simulink model "uz_pmsm_model_old_commit"  (R2023b)
settings: Solver=FixedStepAuto  StartTime=0.0  StopTime=0.05  RelTol=1e-3
PreLoadFcn:
  | uz_pmsm_model_init_parameter
PostLoadFcn:
  | % Import the data from Excel for a lookup table
  | FluxMapData = readtable('C:\Users\Philipp\ultrazohm\ultrazohm_sw\ip_cores\uz_pmsm_model\FluxMapData_2023-05-26_13-07-57.csv');
  | % Row indices for lookup table
  | d_current_in_d_axis = FluxMapData(8:27,1:end);
  | % Column indices for lookup table
  | q_current_in_d_axis = FluxMapData(29:48,1:end);
  | % Output values for lookup table
  | d_Flux_d_axis = FluxMapData(50:69,1:end);
values from neighbouring files (symbols this model uses):
  ad1 = ad_1(1)    [LUT_approx_methode2a.m]    (also in LUT_approx_methode2a_clean.m = ad_self(1); LUT_approx_methode_2a_FEM.m; fitting_parameter.mat = 0.03048394862; fitting_parameter_48V_SynRM.mat = 0.0218446789236)
  ad2 = ad_1(2)    [LUT_approx_methode2a.m]    (also in LUT_approx_methode2a_clean.m = ad_self(2); LUT_approx_methode_2a_FEM.m; fitting_parameter.mat = 0.0402440194669; fitting_parameter_48V_SynRM.mat = 0.015691946268)
  ad3 = ad_1(3)    [LUT_approx_methode2a.m]    (also in LUT_approx_methode2a_clean.m = ad_self(3); LUT_approx_methode_2a_FEM.m; fitting_parameter.mat = -16.4812001193; fitting_parameter_48V_SynRM.mat = 2.77465564774)
  ad4 = ad_3_6(1)    [LUT_approx_methode2a.m]    (also in LUT_approx_methode2a_clean.m = ad_4_6(1); LUT_approx_methode_2a_FEM.m; fitting_parameter.mat = 1.2964378241; fitting_parameter_48V_SynRM.mat = 0.0214529395212)
  ad5 = ad_3_6(2)    [LUT_approx_methode2a.m]    (also in LUT_approx_methode2a_clean.m = ad_4_6(2); LUT_approx_methode_2a_FEM.m; fitting_parameter.mat = 0.000618316734858; fitting_parameter_48V_SynRM.mat = 0.0128514742508)
  ad6 = ad_3_6(3)    [LUT_approx_methode2a.m]    (also in LUT_approx_methode2a_clean.m = ad_4_6(3); LUT_approx_methode_2a_FEM.m; fitting_parameter.mat = -12.2755860444; fitting_parameter_48V_SynRM.mat = 2.54408267654)
  aq1 = aq_1(1)    [LUT_approx_methode2a.m]    (also in LUT_approx_methode2a_clean.m = aq_self(1); LUT_approx_methode_2a_FEM.m; fitting_parameter.mat = 0.0048166705291; fitting_parameter_48V_SynRM.mat = 0.00205546577039)
  aq2 = aq_1(2)    [LUT_approx_methode2a.m]    (also in LUT_approx_methode2a_clean.m = aq_self(2); LUT_approx_methode_2a_FEM.m; fitting_parameter.mat = 0.171595255564; fitting_parameter_48V_SynRM.mat = 0.0602932843871)
  aq3 = aq_1(3)    [LUT_approx_methode2a.m]    (also in LUT_approx_methode2a_clean.m = aq_self(3); LUT_approx_methode_2a_FEM.m; fitting_parameter.mat = 0.000926293864031; fitting_parameter_48V_SynRM.mat = 4.42738872822e-05)
  aq4 = aq_3_6(1)    [LUT_approx_methode2a.m]    (also in LUT_approx_methode2a_clean.m = aq_4_6(1); LUT_approx_methode_2a_FEM.m; fitting_parameter.mat = 0.00500187099075; fitting_parameter_48V_SynRM.mat = 0.000698420875152)
  aq5 = aq_3_6(2)    [LUT_approx_methode2a.m]    (also in LUT_approx_methode2a_clean.m = aq_4_6(2); LUT_approx_methode_2a_FEM.m; fitting_parameter.mat = 0.17052123489; fitting_parameter_48V_SynRM.mat = 0.0493122483219)
  aq6 = aq_3_6(3)    [LUT_approx_methode2a.m]    (also in LUT_approx_methode2a_clean.m = aq_4_6(3); LUT_approx_methode_2a_FEM.m; fitting_parameter.mat = 0.00091860845; fitting_parameter_48V_SynRM.mat = 4.14644316065e-05)
  d_current_d_Flux = FluxMapData{1,1:20}    [uz_pmsm_model_init_parameter.m]
  d_current_q_Flux = FluxMapData{66,1:20}    [uz_pmsm_model_init_parameter.m]
  entkopplung_dynamic = false    [compare_simulation_to_measurement.m]    (also in uz_pmsm_model_init_parameter.m; uz_pmsm_model_init_parameter_clean.m)
  entkopplung_linear = true    [compare_simulation_to_measurement.m]    (also in uz_pmsm_model_init_parameter.m = false; uz_pmsm_model_init_parameter_clean.m = false)
  entkopplung_static = false    [compare_simulation_to_measurement.m]    (also in uz_pmsm_model_init_parameter.m = true; uz_pmsm_model_init_parameter_clean.m)
  Fid1_Giq1 = ((1/2).*(aq3-aq6).*((q_current_set).^2))+((aq1./aq2).*log(cosh(aq2.*q_current_set)))-((aq4/aq5).*log(cosh(aq5.*q_current_set)))    [LUT_approx_methode2a.m]    (also in LUT_approx_methode2a_clean.m; LUT_approx_methode_2a_FEM.m = (1/2).*(aq3-aq6).*((q_current_set).^2)+((aq1./aq2).*log(cosh; fitting_parameter.mat = -0.00135679401385; fitting_parameter_48V_SynRM.mat = 0.221350145237)
  Fid2_Giq2 = ((ad1./ad2).*(log(cosh(ad2.*(d_current_set-ad3))))) - ((ad4./ad5).*(log(cosh(ad5.*(d_current_set-ad6)))))    [LUT_approx_methode2a.m]    (also in LUT_approx_methode2a_clean.m; LUT_approx_methode_2a_FEM.m = ((ad1./ad2).*(log(cosh(ad2.*(d_current_set-ad3))))) - (((ad1; fitting_parameter.mat = 0.0788137932988; fitting_parameter_48V_SynRM.mat = 0.221214979406)
  Flux_d = FluxMapData{43:62,1:20}'*(1e-3)    [uz_pmsm_model_init_parameter.m]
  Flux_q = FluxMapData{108:127,1:20}'*(1e-3)    [uz_pmsm_model_init_parameter.m]
  friction_coefficient = 0.001    [uz_pmsm_model_init_parameter.m]    (also in uz_pmsm_model_init_parameter_clean.m)
  inertia = 0.000084    (= 8.4e-05)    [uz_pmsm_model_init_parameter.m]    (also in uz_pmsm_model_init_parameter_clean.m)
  L_d = 0.3    [uz_pmsm_model_init_parameter.m]    (also in uz_pmsm_model_init_parameter_clean.m = 0.00045)
  L_q = 0.3    [uz_pmsm_model_init_parameter.m]    (also in uz_pmsm_model_init_parameter_clean.m = 0.002)
  load_torque = 0    [uz_pmsm_model_init_parameter.m]
  parameter_nachfuerung = false    [compare_simulation_to_measurement.m]    (also in uz_pmsm_model_init_parameter.m; uz_pmsm_model_init_parameter_clean.m)
  polepair = 4    [uz_pmsm_model_init_parameter.m]    (also in uz_pmsm_model_init_parameter_clean.m)
  praediktion_entkopplung_nonlinear = false    [compare_simulation_to_measurement.m]    (also in uz_pmsm_model_init_parameter.m; uz_pmsm_model_init_parameter_clean.m = true)
  psi_pm = 0.0075    [uz_pmsm_model_init_parameter.m]    (also in uz_pmsm_model_init_parameter_clean.m = 0.0194)
  q_current_d_Flux = FluxMapData{22:41,1}    [uz_pmsm_model_init_parameter.m]
  q_current_q_Flux = FluxMapData{87:106,1}    [uz_pmsm_model_init_parameter.m]
  R_1 = 0.08    [uz_pmsm_model_init_parameter.m]    (also in uz_pmsm_model_init_parameter_clean.m = 0.3)
  rpm = 1250    [uz_pmsm_model_init_parameter.m]
  setpoint_step = 4.0    (= 4)    [compare_simulation_to_measurement.m]    (also in export_csv.m = 10; iae_von_cil_measurements.m = 8; uz_pmsm_model_init_parameter.m = 8; uz_pmsm_model_init_parameter_clean.m = 10)
  simulate_mechanical = true    [compare_simulation_to_measurement.m]    (also in export_csv.m = false; uz_pmsm_model_init_parameter.m = false; uz_pmsm_model_init_parameter_clean.m = false)
  simulate_nonlinear_modell = false    [compare_simulation_to_measurement.m]    (also in uz_pmsm_model_init_parameter.m = true; uz_pmsm_model_init_parameter_clean.m = true)
  simulate_open_loop = true    [compare_simulation_to_measurement.m]    (also in export_csv.m; uz_pmsm_model_init_parameter.m = false; uz_pmsm_model_init_parameter_clean.m = false)
  static_friction_torque = 0.01    [uz_pmsm_model_init_parameter.m]    (also in uz_pmsm_model_init_parameter_clean.m)
  tau_sum = 2*ts_regler    (= 0.0001)    [uz_pmsm_model_init_parameter.m]    (also in uz_pmsm_model_init_parameter_clean.m = 8e-05)
  ts = logs{k}.Values    [export_csv.m]    (also in uz_pmsm_model_init_parameter.m = 2e-06; uz_pmsm_model_init_parameter_clean.m = 2e-06)
  ts_regler = 1/20e3    (= 5e-05)    [uz_pmsm_model_init_parameter.m]    (also in uz_pmsm_model_init_parameter_clean.m = 4e-05)
undefined symbols (not defined in the file or in its folder): Ki_Bo_d, Ki_Bo_q, Kp_Bo_d, Kp_Bo_q, Ldq
libraries: slpidlib x6
(part 2 of 5)

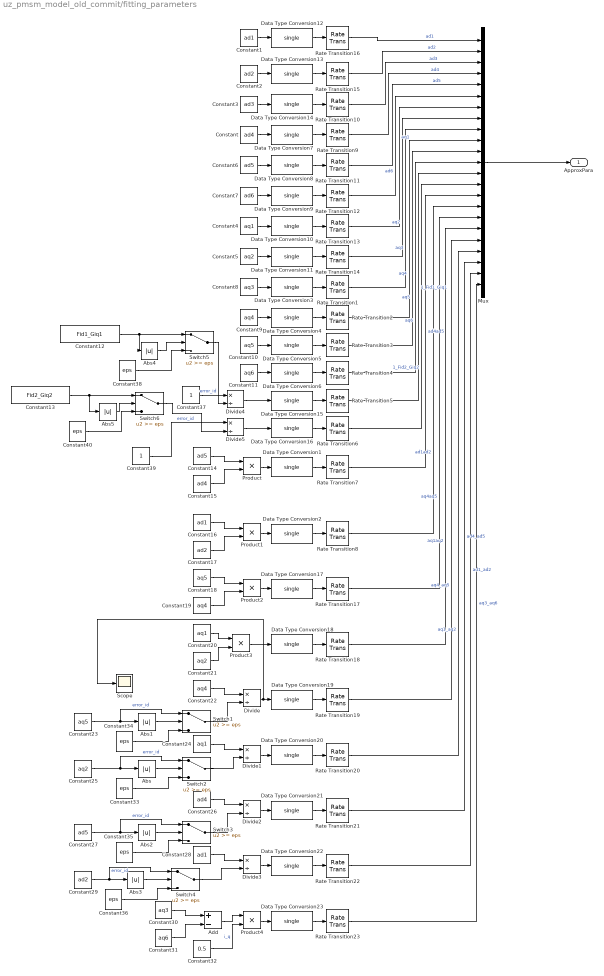
== system uz_pmsm_model_old_commit/fitting_parameters ==
  Abs{,1..5} (6 alike) : Abs  SaturateOnIntegerOverflow=off
  Add : Sum  Inputs=+-
  Constant : Constant  Value=ad4
  Constant1 : Constant  Value=ad1
  Constant10 : Constant  Value=aq5
  Constant11 : Constant  Value=aq6
  Constant12 : Constant  Value=Fid1_Giq1
  Constant13 : Constant  Value=Fid2_Giq2
  Constant14 : Constant  Value=ad5
  Constant15 : Constant  Value=ad4
  Constant16 : Constant  Value=ad1
  Constant17 : Constant  Value=ad2
  Constant18 : Constant  Value=aq5
  Constant19 : Constant  Value=aq4
  Constant2 : Constant  Value=ad2
  Constant20 : Constant  Value=aq1
  Constant21 : Constant  Value=aq2
  Constant22 : Constant  Value=aq4
  Constant23 : Constant  Value=aq5
  Constant24 : Constant  Value=aq1
  Constant25 : Constant  Value=aq2
  Constant26 : Constant  Value=ad4
  Constant27 : Constant  Value=ad5
  Constant28 : Constant  Value=ad1
  Constant29 : Constant  Value=ad2
  Constant3 : Constant  Value=ad3
  Constant30 : Constant  Value=aq3
  Constant31 : Constant  Value=aq6
  Constant32 : Constant  Value=0.5  OutDataTypeStr=double  SampleTime=-1
  Constant{33..36,38,40} (6 alike) : Constant  Value=eps  SampleTime=ts_regler
  Constant37 : Constant
  Constant39 : Constant
  Constant4 : Constant  Value=aq1
  Constant5 : Constant  Value=aq2
  Constant6 : Constant  Value=ad5
  Constant7 : Constant  Value=ad6
  Constant8 : Constant  Value=aq3
  Constant9 : Constant  Value=aq4
  Data Type Conversion{1..23} (23 alike) : DataTypeConversion  OutDataTypeStr=single  SaturateOnIntegerOverflow=off  RndMeth=Floor
  Divide{,1..5} (6 alike) : Product  Inputs=*/
  Mux : Mux  Inputs=23
  Product{,1..4} (5 alike) : Product
  Rate Transition{1..23} (23 alike) : RateTransition  OutPortSampleTime=ts
  Scope : Scope
  Switch{1..6} (6 alike) : Switch  Threshold=eps  SaturateOnIntegerOverflow=off  InputSameDT=off
  ApproxPara : Outport
  wires:
  Constant1/1 -> Data Type Conversion12/1
  Constant/1 -> Data Type Conversion7/1
  Rate Transition10/1 -> Mux/3  "ad3"
  Rate Transition14/1 -> Mux/8  "aq2"
  Constant3/1 -> Data Type Conversion14/1
  Rate Transition12/1 -> Mux/6  "ad6"
  Rate Transition16/1 -> Mux/1  "ad1"
  Rate Transition13/1 -> Mux/7  "aq1"
  Constant5/1 -> Data Type Conversion11/1
  Constant7/1 -> Data Type Conversion9/1
  Rate Transition15/1 -> Mux/2  "ad2"
  Rate Transition9/1 -> Mux/4  "ad4"
  Constant6/1 -> Data Type Conversion8/1
  Constant4/1 -> Data Type Conversion10/1
  Rate Transition11/1 -> Mux/5  "ad5"
  Constant2/1 -> Data Type Conversion13/1
  Rate Transition1/1 -> Mux/9  "aq3"
  Constant8/1 -> Data Type Conversion3/1
  Rate Transition2/1 -> Mux/10  "aq4"
  Constant9/1 -> Data Type Conversion4/1
  Rate Transition3/1 -> Mux/11  "aq5"
  Constant10/1 -> Data Type Conversion5/1
  Rate Transition4/1 -> Mux/12  "aq6"
  Constant11/1 -> Data Type Conversion6/1
  Rate Transition5/1 -> Mux/13  "1_Fid1_Giq1"
  Rate Transition6/1 -> Mux/14  "1_Fid2_Giq2"
  Data Type Conversion11/1 -> Rate Transition14/1
  Data Type Conversion10/1 -> Rate Transition13/1
  Data Type Conversion9/1 -> Rate Transition12/1
  Data Type Conversion12/1 -> Rate Transition16/1
  Data Type Conversion13/1 -> Rate Transition15/1
  Data Type Conversion14/1 -> Rate Transition10/1
  Data Type Conversion7/1 -> Rate Transition9/1
  Data Type Conversion8/1 -> Rate Transition11/1
  Data Type Conversion3/1 -> Rate Transition1/1
  Data Type Conversion4/1 -> Rate Transition2/1
  Data Type Conversion5/1 -> Rate Transition3/1
  Data Type Conversion6/1 -> Rate Transition4/1
  Data Type Conversion15/1 -> Rate Transition5/1
  Data Type Conversion16/1 -> Rate Transition6/1
  Constant14/1 -> Product/1
  Constant15/1 -> Product/2
  Product/1 -> Data Type Conversion1/1
  Data Type Conversion1/1 -> Rate Transition7/1
  Rate Transition7/1 -> Mux/15  "ad4ad5"
  Rate Transition8/1 -> Mux/16  "ad1ad2"
  Constant16/1 -> Product1/1
  Constant17/1 -> Product1/2
  Data Type Conversion2/1 -> Rate Transition8/1
  Product1/1 -> Data Type Conversion2/1
  Constant18/1 -> Product2/1
  Constant19/1 -> Product2/2
  Data Type Conversion17/1 -> Rate Transition17/1
  Product2/1 -> Data Type Conversion17/1
  Rate Transition18/1 -> Mux/18  "aq1aq2"
  Product3/1 -> Data Type Conversion18/1
  Data Type Conversion18/1 -> Rate Transition18/1
  Constant21/1 -> Product3/2
  Constant20/1 -> Product3/1
  Rate Transition17/1 -> Mux/17  "aq4aq5"
  Divide/1 -> Scope/1, Data Type Conversion19/1
  Data Type Conversion19/1 -> Rate Transition19/1
  Constant22/1 -> Divide/1
  Rate Transition19/1 -> Mux/19  "aq4_aq5"
  Constant24/1 -> Divide1/1
  Rate Transition20/1 -> Mux/20  "aq1_aq2"
  Divide1/1 -> Data Type Conversion20/1
  Data Type Conversion20/1 -> Rate Transition20/1
  Data Type Conversion21/1 -> Rate Transition21/1
  Divide2/1 -> Data Type Conversion21/1
  Rate Transition21/1 -> Mux/21  "ad4_ad5"
  Constant26/1 -> Divide2/1
  Constant28/1 -> Divide3/1
  Rate Transition22/1 -> Mux/22  "ad1_ad2"
  Divide3/1 -> Data Type Conversion22/1
  Data Type Conversion22/1 -> Rate Transition22/1
  Data Type Conversion23/1 -> Rate Transition23/1
  Constant30/1 -> Add/1
  Constant31/1 -> Add/2
  Rate Transition23/1 -> Mux/23  "aq3_aq6"
  Product4/1 -> Data Type Conversion23/1
  Constant32/1 -> Product4/2  "i_q"
  Add/1 -> Product4/1
  Mux/1 -> ApproxPara/1
  Constant25/1 -> Switch2/1, Abs/1  "error_id"
  Switch2/1 -> Divide1/2
  Abs/1 -> Switch2/2
  Constant33/1 -> Switch2/3
  Constant23/1 -> Switch1/1, Abs1/1  "error_id"
  Switch1/1 -> Divide/2
  Abs1/1 -> Switch1/2
  Constant34/1 -> Switch1/3
  Constant27/1 -> Switch3/1, Abs2/1  "error_id"
  Switch3/1 -> Divide2/2
  Abs2/1 -> Switch3/2
  Constant35/1 -> Switch3/3
  Constant29/1 -> Switch4/1, Abs3/1  "error_id"
  Switch4/1 -> Divide3/2
  Abs3/1 -> Switch4/2
  Constant36/1 -> Switch4/3
  Abs4/1 -> Switch5/2
  Constant38/1 -> Switch5/3
  Divide4/1 -> Data Type Conversion15/1
  Switch5/1 -> Divide4/2
  Constant12/1 -> Abs4/1, Switch5/1
  Constant37/1 -> Divide4/1  "error_id"
  Constant39/1 -> Divide5/1  "error_id"
  Constant13/1 -> Abs5/1, Switch6/1
  Constant40/1 -> Switch6/3
  Abs5/1 -> Switch6/2
  Divide5/1 -> Data Type Conversion16/1
  Switch6/1 -> Divide5/2

== system uz_pmsm_model_old_commit/model_parameters1 ==
  Bus Creator : BusCreator  Inputs=8
  Constant : Constant  Value=L_d
  Constant6 : Constant  Value=L_q
  Constant7 : Constant  Value=R_1
  Constant8 : Constant  Value=polepair
  Constant9 : Constant  Value=psi_pm
  Data Type Conversion{7..14} (8 alike) : DataTypeConversion  OutDataTypeStr=single  SaturateOnIntegerOverflow=off  RndMeth=Floor
  J : Constant  Value=1/inertia
  M_R0 : Constant  Value=static_friction_torque
  Rate Transition{9..16} (8 alike) : RateTransition  OutPortSampleTime=ts
  mu : Constant  Value=friction_coefficient
  Out1 : Outport
  wires:
  Data Type Conversion12/1 -> Rate Transition16/1
  Data Type Conversion7/1 -> Rate Transition9/1
  Rate Transition10/1 -> Bus Creator/3  "M_R0"
  Rate Transition14/1 -> Bus Creator/8  "psi_pm"
  Data Type Conversion14/1 -> Rate Transition10/1
  Rate Transition12/1 -> Bus Creator/6  "R_1"
  Rate Transition16/1 -> Bus Creator/1  "1_J"
  Rate Transition13/1 -> Bus Creator/7  "polepair"
  Bus Creator/1 -> Out1/1
  Data Type Conversion11/1 -> Rate Transition14/1
  Constant8/1 -> Data Type Conversion10/1
  Data Type Conversion9/1 -> Rate Transition12/1
  Rate Transition15/1 -> Bus Creator/2  "mu"
  Constant6/1 -> Data Type Conversion8/1
  Rate Transition9/1 -> Bus Creator/4  "1_L_d"
  J/1 -> Data Type Conversion12/1
  Data Type Conversion8/1 -> Rate Transition11/1
  Data Type Conversion10/1 -> Rate Transition13/1
  mu/1 -> Data Type Conversion13/1
  M_R0/1 -> Data Type Conversion14/1
  Rate Transition11/1 -> Bus Creator/5  "1_L_q"
  Data Type Conversion13/1 -> Rate Transition15/1
  Constant7/1 -> Data Type Conversion9/1
  Constant9/1 -> Data Type Conversion11/1
  Constant/1 -> Data Type Conversion7/1

== system uz_pmsm_model_old_commit/uz_pmsm_model ==
  reset_integrators : Inport
  simulate_mechanical : Inport  Port=2
  simulate_nonlinear : Inport  Port=3
  reciprocal_J : Inport  Port=4
  mu : Inport  Port=5
  M_n0 : Inport  Port=6
  R1 : Inport  Port=7
  polepairs : Inport  Port=8
  Ld : Inport  Port=9
  Lq : Inport  Port=10
  psi_pm : Inport  Port=11
  fitting_parameter : Inport  Port=12
  inputs : Inport  Port=13
  Demux : Demux
  Mux : Mux
  Switch : Switch  Criteria=u2 ~= 0  SaturateOnIntegerOverflow=off  InputSameDT=off
  Switch1 : Switch  Criteria=u2 ~= 0  SaturateOnIntegerOverflow=off  InputSameDT=off
  mechanical_system : Subsystem
  pmsm : Subsystem
  torque_calculation : Subsystem
  outputs : Outport
  wires:
  reset_integrators/1 -> pmsm/1(reset1), mechanical_system/1(reset)
  Demux/3 -> Switch1/3, Switch/3  "omega_mech"
  Switch/1 -> pmsm/11(omega_mech1)
  pmsm/2(psi_d1) -> torque_calculation/2(psi_d)
  Demux/4 -> mechanical_system/6(load_torque)  "load_torque"
  pmsm/3(psi_q1) -> torque_calculation/3(psi_q)
  Demux/1 -> pmsm/3(u_d1)  "u_d"
  simulate_mechanical/1 -> Switch1/2, Switch/2
  Demux/2 -> pmsm/4(u_q1)  "u_q"
  mechanical_system/1(omega_mech) -> Switch/1, Switch1/1
  pmsm/4(I_q1) -> torque_calculation/5(I_q), Mux/2  "i_q"
  pmsm/1(I_d1) -> Mux/1, torque_calculation/1(I_d)  "i_d"
  Switch1/1 -> Mux/4  "i_q"
  torque_calculation/1(M_Mi) -> mechanical_system/2(M_Mi), Mux/3  "i_q"
  inputs/1 -> Demux/1
  Mux/1 -> outputs/1
  simulate_nonlinear/1 -> pmsm/2(simulate_nonlinear)
  R1/1 -> pmsm/5(R2)
  polepairs/1 -> torque_calculation/4(polepairs), pmsm/6(polepairs1)
  Ld/1 -> pmsm/7(Ld)
  Lq/1 -> pmsm/8(Lq)
  psi_pm/1 -> pmsm/9(psi_pm)
  mu/1 -> mechanical_system/3(mu)
  M_n0/1 -> mechanical_system/4(M_n0)
  reciprocal_J/1 -> mechanical_system/5(reciprocal_J)
  fitting_parameter/1 -> pmsm/10(fitting_parameters)

== system uz_pmsm_model_old_commit/Curren t_Controller_With_FluxMaps_OLD/#embedded-Coder ==
  Psi_d_q : Subsystem
  Reglernachführung2 : Subsystem
  Subsystem : Subsystem
  approximate_flux_d : Subsystem
  approximate_flux_q : Subsystem

== system uz_pmsm_model_old_commit/Curren t_Controller_With_FluxMaps_OLD/Entkopplung_flags ==
  u_d_static : Inport
  u_q_static : Inport  Port=2
  u_d_praed : Inport  Port=3
  u_q_praed : Inport  Port=4
  u_d_lin : Inport  Port=5
  u_q_lin : Inport  Port=6
  u_d_dyn : Inport  Port=7
  u_q_dyn : Inport  Port=8
  0 : Constant  Value=0
  Switch{1..8} (8 alike) : Switch  Criteria=u2 > Threshold  SaturateOnIntegerOverflow=off  InputSameDT=off
  entkopplung_dynamic : Constant  Value=entkopplung_dynamic
  entkopplung_linear : Constant  Value=entkopplung_linear
  entkopplung_preadiktion : Constant  Value=praediktion_entkopplung_nonlinear
  entkopplung_static : Constant  Value=entkopplung_static
  u_d_entk : Outport
  u_q_entk : Outport  Port=2
  wires:
  Switch3/1 -> u_d_entk/1
  Switch4/1 -> Switch2/3
  entkopplung_preadiktion/1 -> Switch2/2, Switch3/2
  Switch1/1 -> Switch3/3
  u_d_praed/1 -> Switch3/1
  Switch2/1 -> u_q_entk/1
  u_q_praed/1 -> Switch2/1
  entkopplung_static/1 -> Switch4/2, Switch1/2
  u_d_static/1 -> Switch1/1
  u_d_lin/1 -> Switch5/1
  Switch5/1 -> Switch1/3
  entkopplung_linear/1 -> Switch6/2, Switch5/2
  entkopplung_dynamic/1 -> Switch8/2, Switch7/2
  0/1 -> Switch8/3, Switch7/3
  Switch6/1 -> Switch4/3
  u_q_static/1 -> Switch4/1
  u_q_lin/1 -> Switch6/1
  u_d_dyn/1 -> Switch7/1
  Switch8/1 -> Switch6/3
  u_q_dyn/1 -> Switch8/1
  Switch7/1 -> Switch5/3

== system uz_pmsm_model_old_commit/Curren t_Controller_With_FluxMaps_OLD/Entkopplungen ==
  u_q : Inport
  u_d : Inport  Port=2
  uq : Inport  Port=3
  ud : Inport  Port=4
  i_d : Inport  Port=5
  psi_d_LUT : Inport  Port=6
  psi_q_LUT : Inport  Port=7
  Ldq_LUT : Inport  Port=8
  Lqd_LUT : Inport  Port=9
  i_q : Inport  Port=10
  omega_m : Inport  Port=11
  Lineare_Entkopplung : Subsystem
  Scope : Scope  NumInputPorts=2
  decoupling_praediktion : Subsystem
  dynamic_nonlinear_entkopplung1 : Subsystem
  static_nonlinear_entkopplung : Subsystem
  u_d_static : Outport
  u_q_static : Outport  Port=2
  u_d_prae : Outport  Port=3
  u_q_prae : Outport  Port=4
  u_d_lin : Outport  Port=5
  u_q_lin : Outport  Port=6
  u_d_dyn : Outport  Port=7
  u_q_dyn1 : Outport  Port=8
  wires:
  psi_d_LUT/1 -> static_nonlinear_entkopplung/1(psi_d), dynamic_nonlinear_entkopplung1/3(psi_d), decoupling_praediktion/9(psi_d)
  omega_m/1 -> dynamic_nonlinear_entkopplung1/7(omega_m), Lineare_Entkopplung/3(omega_m), static_nonlinear_entkopplung/3(omega_m), decoupling_praediktion/5(omega_m)
  psi_q_LUT/1 -> dynamic_nonlinear_entkopplung1/4(psi_q), decoupling_praediktion/8(psi_q), static_nonlinear_entkopplung/2(psi_q)
  u_q/1 -> decoupling_praediktion/4(u_q_1)
  i_d/1 -> dynamic_nonlinear_entkopplung1/1(i_d), Lineare_Entkopplung/1(i_d), decoupling_praediktion/1(i_d)
  i_q/1 -> dynamic_nonlinear_entkopplung1/2(i_q), Lineare_Entkopplung/2(i_q), decoupling_praediktion/3(i_q)
  ud/1 -> decoupling_praediktion/6(u_d_k)
  uq/1 -> decoupling_praediktion/7(u_q_k)
  u_d/1 -> decoupling_praediktion/2(u_d_1)
  static_nonlinear_entkopplung/1(u_d) -> u_d_static/1
  Lineare_Entkopplung/1(u_d) -> Scope/1, u_d_lin/1
  static_nonlinear_entkopplung/2(u_q) -> u_q_static/1
  decoupling_praediktion/1(u_d_entk) -> u_d_prae/1
  Lineare_Entkopplung/2(u_q) -> Scope/2, u_q_lin/1
  decoupling_praediktion/2(u_q_entk) -> u_q_prae/1
  dynamic_nonlinear_entkopplung1/1(u_d) -> u_d_dyn/1
  dynamic_nonlinear_entkopplung1/2(u_q) -> u_q_dyn1/1
  Ldq_LUT/1 -> dynamic_nonlinear_entkopplung1/5(Ldq_LUT)
  Lqd_LUT/1 -> dynamic_nonlinear_entkopplung1/6(Lqd_LUT)

== system uz_pmsm_model_old_commit/Curren t_Controller_With_FluxMaps_OLD/Psi_d_q ==
  I_d_set : Inport
  I_d : Inport  Port=2
  I_q_set : Inport  Port=3
  I_q : Inport  Port=4
  ApproxPara : Inport  Port=5
  Constant4 : Constant  Value="eps(\"single\")"  SampleTime=ts_regler
  Constant5 : Constant  Value="eps(\"single\")"  SampleTime=ts_regler
  Data Type Conversion{1..5} (5 alike) : DataTypeConversion  OutDataTypeStr=single  SaturateOnIntegerOverflow=off  RndMeth=Floor
  Divide : Product  Inputs=*/
  Divide1 : Product  Inputs=*/
  Scope : Scope  NumInputPorts=4
  Sum{1..2,4..5} (4 alike) : Sum  Inputs=|+-
  Switch2 : Switch  Criteria=u2 ~= 0  Threshold=eps  SaturateOnIntegerOverflow=off  InputSameDT=off
  Switch3 : Switch  Criteria=u2 ~= 0  Threshold=eps  SaturateOnIntegerOverflow=off  InputSameDT=off
  psid_approx : Subsystem
  psid_approx1 : Subsystem
  psiq_approx : Subsystem
  psiq_approx1 : Subsystem
  Ldd_approx : Outport
  Lqq_approx : Outport  Port=2
  psid : Outport  Port=3
  psiq : Outport  Port=4
  wires:
  I_q/1 -> Data Type Conversion4/1
  psid_approx/1(psid) -> Scope/3, Sum4/1  "psi_d_set"
  psiq_approx/1(psiq) -> Scope/4, Sum5/1  "psi_q_set"
  ApproxPara/1 -> Data Type Conversion5/1
  I_d/1 -> Data Type Conversion2/1
  psiq_approx1/1(psiq) -> Scope/1, psiq/1, Sum5/2  "psi_q"
  psid_approx1/1(psid) -> Scope/2, psid/1, Sum4/2  "psi_d"
  Constant5/1 -> Switch3/3
  Switch2/1 -> Divide/2
  Switch3/1 -> Divide1/2
  Divide/1 -> Ldd_approx/1  "Ldd_approx"
  Divide1/1 -> Lqq_approx/1  "Lqq_approx"
  Constant4/1 -> Switch2/3
  Sum5/1 -> Divide1/1
  Sum4/1 -> Divide/1
  Sum2/1 -> Switch2/2, Switch2/1
  I_q_set/1 -> Data Type Conversion3/1
  I_d_set/1 -> Data Type Conversion1/1
  Sum1/1 -> Switch3/2, Switch3/1
  Data Type Conversion1/1 -> psid_approx/1(Id), Sum2/1  "omega_mech"
  Data Type Conversion3/1 -> Sum1/1, psiq_approx/2(Iq)  "omega_mech"
  Data Type Conversion2/1 -> psid_approx1/1(Id), psiq_approx1/1(Id), Sum2/2, psiq_approx/1(Id)  "omega_mech"
  Data Type Conversion4/1 -> Sum1/2, psiq_approx1/2(Iq), psid_approx1/2(Iq), psid_approx/2(Iq)  "omega_mech"
  Data Type Conversion5/1 -> psid_approx1/3(FittingParameters), psid_approx/3(FittingParameters), psiq_approx/3(FittingParameters), psiq_approx1/3(FittingParameters)  "omega_mech"

== system uz_pmsm_model_old_commit/Curren t_Controller_With_FluxMaps_OLD/Psi_d_q1 ==
  I_d : Inport
  I_q : Inport  Port=2
  ApproxPara : Inport  Port=3
  Ldd_approx1 : Subsystem
  Lqq_approx1 : Subsystem
  psid_approx : Subsystem
  psiq_approx : Subsystem
  psi_d : Outport
  Ldd : Outport  Port=2
  psi_q : Outport  Port=3
  Lqq : Outport  Port=4
  wires:
  psid_approx/1(psid) -> psi_d/1  "psi_d"
  psiq_approx/1(psiq) -> psi_q/1  "psi_q"
  I_q/1 -> psid_approx/2(Iq), Lqq_approx1/2(Iq), psiq_approx/2(Iq)
  psid_approx/2(psiq_cross_s1_integrated) -> Ldd_approx1/1(psiq_cross_s1_integrated)
  I_d/1 -> Ldd_approx1/2(Id), psid_approx/1(Id), psiq_approx/1(Id)
  psiq_approx/2(psid_cross_s1_integrated) -> Lqq_approx1/1(psid_cross_s1_integrated)
  Ldd_approx1/1(Ldd) -> Ldd/1  "Ldd"
  Lqq_approx1/1(Lqq) -> Lqq/1  "Lqq"
  ApproxPara/1 -> psiq_approx/3(FittingParameters), Ldd_approx1/3(FittingParameters), psid_approx/3(FittingParameters), Lqq_approx1/3(FittingParameters)

== system uz_pmsm_model_old_commit/Curren t_Controller_With_FluxMaps_OLD/Psi_d_q2 ==
  I_d_set : Inport
  I_d : Inport  Port=2
  I_q_set : Inport  Port=3
  I_q : Inport  Port=4
  ApproxPara : Inport  Port=5
  Ldd_approx1 : Subsystem
  Lqq_approx1 : Subsystem
  Scope : Scope  NumInputPorts=3
  psid_approx : Subsystem
  psid_approx1 : Subsystem
  psiq_approx : Subsystem
  psiq_approx1 : Subsystem
  psi_d_set : Outport
  psi_q_set : Outport  Port=2
  psi_d_LUT : Outport  Port=3
  psi_q_LUT : Outport  Port=4
  Lqq : Outport  Port=5
  Ldd : Outport  Port=6
  wires:
  I_q/1 -> Lqq_approx1/2(Iq), psiq_approx1/2(Iq), psid_approx1/2(Iq), psid_approx/2(Iq)
  psid_approx/1(psid) -> psi_d_set/1  "psi_d"
  psiq_approx/1(psiq) -> psi_q_set/1  "psi_q"
  ApproxPara/1 -> Ldd_approx1/3(FittingParameters), Lqq_approx1/3(FittingParameters), psiq_approx1/3(FittingParameters), psid_approx/3(FittingParameters), psid_approx1/3(FittingParameters), psiq_approx/3(FittingParameters)
  I_q_set/1 -> psiq_approx/2(Iq)
  I_d_set/1 -> psid_approx/1(Id)
  I_d/1 -> psiq_approx/1(Id), Ldd_approx1/2(Id), psiq_approx1/1(Id), psid_approx1/1(Id)
  psiq_approx1/1(psiq) -> Scope/1, psi_q_LUT/1  "psi_q_test"
  psid_approx1/1(psid) -> psi_d_LUT/1  "psi_d"
  Ldd_approx1/1(Ldd) -> Ldd/1  "Ldd_test"
  Lqq_approx1/1(Lqq) -> Scope/3, Lqq/1  "Lqq_test"
  psiq_approx1/2(psid_cross_s1_integrated) -> Lqq_approx1/1(psid_cross_s1_integrated), Scope/2  "psid_cross_rück_test"
  psid_approx1/2(psiq_cross_s1_integrated) -> Ldd_approx1/1(psiq_cross_s1_integrated)

== system uz_pmsm_model_old_commit/Curren t_Controller_With_FluxMaps_OLD/Reglernachführung ==
  Flag : Inport
  deadtime : Inport  Port=2
  R_s : Inport  Port=3
  Ld : Inport  Port=4
  Lq : Inport  Port=5
  Ldd : Inport  Port=6
  Lqq : Inport  Port=7
  Product{,1..4} (5 alike) : Product
  Scope : Scope  NumInputPorts=2
  Switch : Switch  Criteria=u2 > Threshold  SaturateOnIntegerOverflow=off  InputSameDT=off
  Switch1 : Switch  Criteria=u2 > Threshold  SaturateOnIntegerOverflow=off  InputSameDT=off
  K_p_d : Outport
  K_p_q : Outport  Port=2
  K_I : Outport  Port=3
  wires:
  Product/1 -> K_p_d/1
  Product1/1 -> K_p_q/1
  Product2/1 -> K_I/1
  deadtime/1 -> Product3/2, Product4/2, Product/2, Product2/1, Product1/1
  R_s/1 -> Product2/2  "id_regler"
  Flag/1 -> Switch/2, Switch1/2
  Ld/1 -> Switch/3
  Switch/1 -> Product/1
  Lq/1 -> Switch1/3
  Switch1/1 -> Product1/2
  Ldd/1 -> Switch/1, Product3/1
  Product3/1 -> Scope/1  "Kp_d_adap"
  Lqq/1 -> Product4/1, Switch1/1  "id_regler"
  Product4/1 -> Scope/2  "Kp_q_adap"

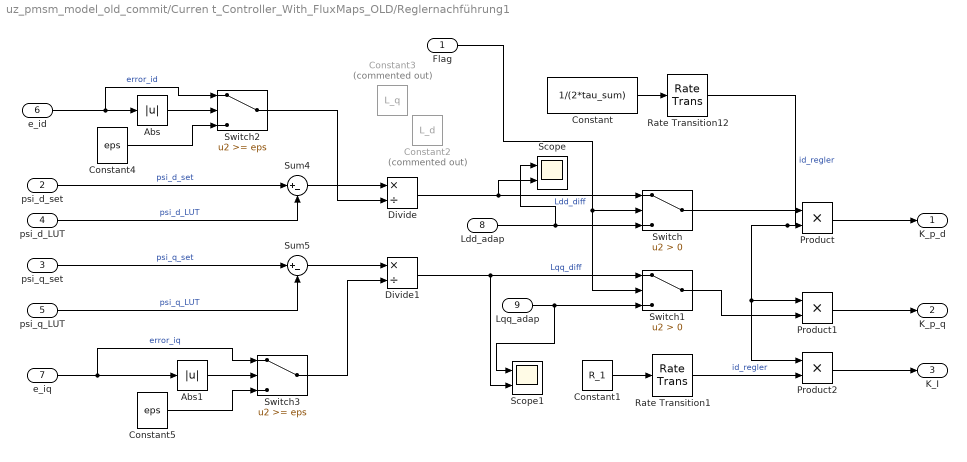
== system uz_pmsm_model_old_commit/Curren t_Controller_With_FluxMaps_OLD/Reglernachführung1 ==
  Flag : Inport
  psi_d_set : Inport  Port=2
  psi_q_set : Inport  Port=3
  psi_d_LUT : Inport  Port=4
  psi_q_LUT : Inport  Port=5
  e_id : Inport  Port=6
  e_iq : Inport  Port=7
  Ldd_adap : Inport  Port=8
  Lqq_adap : Inport  Port=9
  Abs : Abs  SaturateOnIntegerOverflow=off
  Abs1 : Abs  SaturateOnIntegerOverflow=off
  Constant : Constant  Value=1/(2*tau_sum)
  Constant1 : Constant  Value=R_1
  Constant2 : Constant  Commented=on  Value=L_d
  Constant3 : Constant  Commented=on  Value=L_q
  Constant4 : Constant  Value=eps  SampleTime=ts_regler
  Constant5 : Constant  Value=eps  SampleTime=ts_regler
  Divide : Product  Inputs=*/
  Divide1 : Product  Inputs=*/
  Product : Product
  Product1 : Product
  Product2 : Product
  Rate Transition1 : RateTransition  OutPortSampleTime=ts_regler
  Rate Transition12 : RateTransition  OutPortSampleTime=ts_regler
  Scope : Scope  NumInputPorts=2
  Scope1 : Scope  NumInputPorts=2
  Sum4 : Sum  Inputs=|+-
  Sum5 : Sum  Inputs=|+-
  Switch : Switch  Criteria=u2 > Threshold  SaturateOnIntegerOverflow=off  InputSameDT=off
  Switch1 : Switch  Criteria=u2 > Threshold  SaturateOnIntegerOverflow=off  InputSameDT=off
  Switch2 : Switch  Threshold=eps  SaturateOnIntegerOverflow=off  InputSameDT=off
  Switch3 : Switch  Threshold=eps  SaturateOnIntegerOverflow=off  InputSameDT=off
  K_p_d : Outport
  K_p_q : Outport  Port=2
  K_I : Outport  Port=3
  wires:
  Constant/1 -> Rate Transition12/1
  Product/1 -> K_p_d/1
  Product1/1 -> K_p_q/1
  Product2/1 -> K_I/1
  Constant1/1 -> Rate Transition1/1
  Rate Transition12/1 -> Product2/1, Product1/1, Product/2  "id_regler"
  Rate Transition1/1 -> Product2/2  "id_regler"
  Flag/1 -> Switch/2, Switch1/2
  Ldd_adap/1 -> Scope/1, Switch/3
  Switch/1 -> Product/1
  Lqq_adap/1 -> Scope1/1, Switch1/3
  Switch1/1 -> Product1/2
  Sum4/1 -> Divide/1
  psi_q_LUT/1 -> Sum5/2  "psi_q_LUT"
  Sum5/1 -> Divide1/1
  psi_d_LUT/1 -> Sum4/2  "psi_d_LUT"
  psi_d_set/1 -> Sum4/1  "psi_d_set"
  psi_q_set/1 -> Sum5/1  "psi_q_set"
  Divide/1 -> Scope/2, Switch/1  "Ldd_diff"
  Divide1/1 -> Scope1/2, Switch1/1  "Lqq_diff"
  e_id/1 -> Switch2/1, Abs/1  "error_id"
  Constant4/1 -> Switch2/3
  Abs/1 -> Switch2/2
  Switch2/1 -> Divide/2
  e_iq/1 -> Switch3/1, Abs1/1  "error_iq"
  Switch3/1 -> Divide1/2
  Abs1/1 -> Switch3/2
  Constant5/1 -> Switch3/3

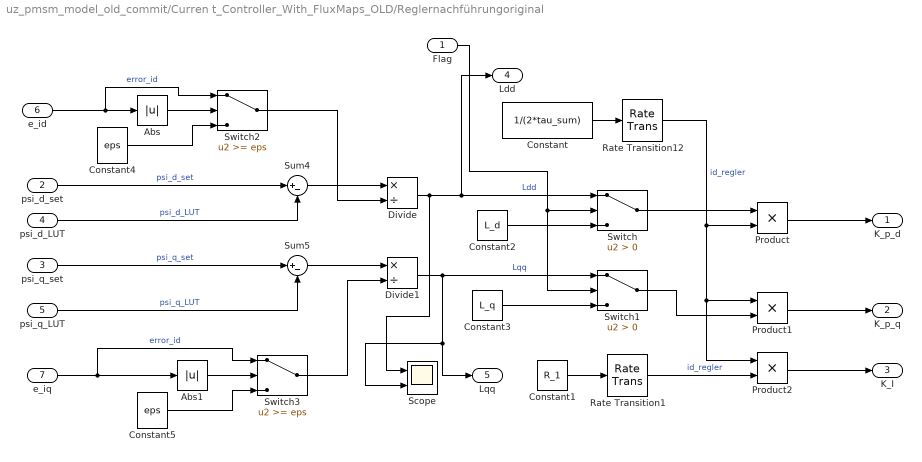
== system uz_pmsm_model_old_commit/Curren t_Controller_With_FluxMaps_OLD/Reglernachführungoriginal ==
  Flag : Inport
  psi_d_set : Inport  Port=2
  psi_q_set : Inport  Port=3
  psi_d_LUT : Inport  Port=4
  psi_q_LUT : Inport  Port=5
  e_id : Inport  Port=6
  e_iq : Inport  Port=7
  Abs : Abs  SaturateOnIntegerOverflow=off
  Abs1 : Abs  SaturateOnIntegerOverflow=off
  Constant : Constant  Value=1/(2*tau_sum)
  Constant1 : Constant  Value=R_1
  Constant2 : Constant  Value=L_d
  Constant3 : Constant  Value=L_q
  Constant4 : Constant  Value=eps  SampleTime=ts_regler
  Constant5 : Constant  Value=eps  SampleTime=ts_regler
  Divide : Product  Inputs=*/
  Divide1 : Product  Inputs=*/
  Product : Product
  Product1 : Product
  Product2 : Product
  Rate Transition1 : RateTransition  OutPortSampleTime=ts_regler
  Rate Transition12 : RateTransition  OutPortSampleTime=ts_regler
  Scope : Scope  NumInputPorts=2
  Sum4 : Sum  Inputs=|+-
  Sum5 : Sum  Inputs=|+-
  Switch : Switch  Criteria=u2 > Threshold  SaturateOnIntegerOverflow=off  InputSameDT=off
  Switch1 : Switch  Criteria=u2 > Threshold  SaturateOnIntegerOverflow=off  InputSameDT=off
  Switch2 : Switch  Threshold=eps  SaturateOnIntegerOverflow=off  InputSameDT=off
  Switch3 : Switch  Threshold=eps  SaturateOnIntegerOverflow=off  InputSameDT=off
  K_p_d : Outport
  K_p_q : Outport  Port=2
  K_I : Outport  Port=3
  Ldd : Outport  Port=4
  Lqq : Outport  Port=5
  wires:
  Constant/1 -> Rate Transition12/1
  Product/1 -> K_p_d/1
  Product1/1 -> K_p_q/1
  Product2/1 -> K_I/1
  Constant1/1 -> Rate Transition1/1
  Rate Transition12/1 -> Product2/1, Product1/1, Product/2  "id_regler"
  Rate Transition1/1 -> Product2/2  "id_regler"
  Flag/1 -> Switch/2, Switch1/2
  Constant2/1 -> Switch/3
  Switch/1 -> Product/1
  Constant3/1 -> Switch1/3
  Switch1/1 -> Product1/2
  Sum4/1 -> Divide/1
  psi_q_LUT/1 -> Sum5/2  "psi_q_LUT"
  Sum5/1 -> Divide1/1
  psi_d_LUT/1 -> Sum4/2  "psi_d_LUT"
  psi_d_set/1 -> Sum4/1  "psi_d_set"
  psi_q_set/1 -> Sum5/1  "psi_q_set"
  Divide/1 -> Scope/1, Ldd/1, Switch/1  "Ldd"
  Divide1/1 -> Scope/2, Lqq/1, Switch1/1  "Lqq"
  e_id/1 -> Switch2/1, Abs/1  "error_id"
  Constant4/1 -> Switch2/3
  Abs/1 -> Switch2/2
  Switch2/1 -> Divide/2
  e_iq/1 -> Switch3/1, Abs1/1  "error_id"
  Switch3/1 -> Divide1/2
  Abs1/1 -> Switch3/2
  Constant5/1 -> Switch3/3

== system uz_pmsm_model_old_commit/Current_Controller1/Entkopplung_flags ==
  u_d_static : Inport
  u_q_static : Inport  Port=2
  u_d_praed : Inport  Port=3
  u_q_praed : Inport  Port=4
  u_d_lin : Inport  Port=5
  u_q_lin : Inport  Port=6
  u_d_dyn : Inport  Port=7
  u_q_dyn : Inport  Port=8
  0 : Constant  Value=0
  Switch{1..8} (8 alike) : Switch  Criteria=u2 > Threshold  SaturateOnIntegerOverflow=off  InputSameDT=off
  entkopplung_dynamic : Constant  Value=entkopplung_dynamic
  entkopplung_linear : Constant  Value=entkopplung_linear
  entkopplung_preadiktion : Constant  Value=praediktion_entkopplung_nonlinear
  entkopplung_static : Constant  Value=entkopplung_static
  u_d_entk : Outport
  u_q_entk : Outport  Port=2
  wires:
  Switch3/1 -> u_d_entk/1
  Switch4/1 -> Switch2/3
  entkopplung_preadiktion/1 -> Switch2/2, Switch3/2
  Switch1/1 -> Switch3/3
  u_d_praed/1 -> Switch3/1
  Switch2/1 -> u_q_entk/1
  u_q_praed/1 -> Switch2/1
  entkopplung_static/1 -> Switch4/2, Switch1/2
  u_d_static/1 -> Switch1/1
  u_d_lin/1 -> Switch5/1
  Switch5/1 -> Switch1/3
  entkopplung_linear/1 -> Switch6/2, Switch5/2
  entkopplung_dynamic/1 -> Switch8/2, Switch7/2
  0/1 -> Switch8/3, Switch7/3
  Switch6/1 -> Switch4/3
  u_q_static/1 -> Switch4/1
  u_q_lin/1 -> Switch6/1
  u_d_dyn/1 -> Switch7/1
  Switch8/1 -> Switch6/3
  u_q_dyn/1 -> Switch8/1
  Switch7/1 -> Switch5/3

== system uz_pmsm_model_old_commit/Current_Controller1/Entkopplungen ==
  u_q : Inport
  u_d : Inport  Port=2
  uq : Inport  Port=3
  ud : Inport  Port=4
  i_d : Inport  Port=5
  psi_d_LUT : Inport  Port=6
  psi_q_LUT : Inport  Port=7
  Ldq_LUT : Inport  Port=8
  Lqd_LUT : Inport  Port=9
  i_q : Inport  Port=10
  omega_m : Inport  Port=11
  Lineare_Entkopplung : Subsystem
  decoupling_praediktion : Subsystem
  dynamic_nonlinear_entkopplung1 : Subsystem  Commented=on
  static_nonlinear_entkopplung : Subsystem
  u_d_static : Outport
  u_q_static : Outport  Port=2
  u_d_prae : Outport  Port=3
  u_q_prae : Outport  Port=4
  u_d_lin : Outport  Port=5
  u_q_lin : Outport  Port=6
  u_d_dyn : Outport  Port=7
  u_q_dyn1 : Outport  Port=8
  wires:
  psi_d_LUT/1 -> static_nonlinear_entkopplung/1(psi_d), dynamic_nonlinear_entkopplung1/3(psi_d), decoupling_praediktion/9(psi_d)
  omega_m/1 -> dynamic_nonlinear_entkopplung1/7(omega_m), Lineare_Entkopplung/3(omega_m), static_nonlinear_entkopplung/3(omega_m), decoupling_praediktion/5(omega_m)
  psi_q_LUT/1 -> dynamic_nonlinear_entkopplung1/4(psi_q), decoupling_praediktion/8(psi_q), static_nonlinear_entkopplung/2(psi_q)
  u_q/1 -> decoupling_praediktion/4(u_q_1)
  i_d/1 -> dynamic_nonlinear_entkopplung1/1(i_d), Lineare_Entkopplung/1(i_d), decoupling_praediktion/1(i_d)
  i_q/1 -> dynamic_nonlinear_entkopplung1/2(i_q), Lineare_Entkopplung/2(i_q), decoupling_praediktion/3(i_q)
  ud/1 -> decoupling_praediktion/6(u_d_k)
  uq/1 -> decoupling_praediktion/7(u_q_k)
  u_d/1 -> decoupling_praediktion/2(u_d_1)
  static_nonlinear_entkopplung/1(u_d) -> u_d_static/1
  Lineare_Entkopplung/1(u_d) -> u_d_lin/1
  static_nonlinear_entkopplung/2(u_q) -> u_q_static/1
  decoupling_praediktion/1(u_d_entk) -> u_d_prae/1
  Lineare_Entkopplung/2(u_q) -> u_q_lin/1
  decoupling_praediktion/2(u_q_entk) -> u_q_prae/1
  dynamic_nonlinear_entkopplung1/1(u_d) -> u_d_dyn/1
  dynamic_nonlinear_entkopplung1/2(u_q) -> u_q_dyn1/1
  Ldq_LUT/1 -> dynamic_nonlinear_entkopplung1/5(Ldq_LUT)
  Lqd_LUT/1 -> dynamic_nonlinear_entkopplung1/6(Lqd_LUT)

== system uz_pmsm_model_old_commit/Current_Controller1/Psi_d_q1 ==
  I_d : Inport
  I_q : Inport  Port=2
  ApproxPara : Inport  Port=3
  Ldd_approx1 : Subsystem
  Lqq_approx1 : Subsystem
  psid_approx : Subsystem
  psiq_approx : Subsystem
  psi_d : Outport
  Ldd : Outport  Port=2
  psi_q : Outport  Port=3
  Lqq : Outport  Port=4
  wires:
  psid_approx/1(psid) -> psi_d/1  "psi_d"
  psiq_approx/1(psiq) -> psi_q/1  "psi_q"
  I_q/1 -> psid_approx/2(Iq), Lqq_approx1/2(Iq), psiq_approx/2(Iq)
  psid_approx/2(psiq_cross_s1_integrated) -> Ldd_approx1/1(psiq_cross_s1_integrated)
  I_d/1 -> Ldd_approx1/2(Id), psid_approx/1(Id), psiq_approx/1(Id)
  psiq_approx/2(psid_cross_s1_integrated) -> Lqq_approx1/1(psid_cross_s1_integrated)
  Ldd_approx1/1(Ldd) -> Ldd/1  "Ldd"
  Lqq_approx1/1(Lqq) -> Lqq/1  "Lqq"
  ApproxPara/1 -> psiq_approx/3(FittingParameters), Ldd_approx1/3(FittingParameters), psid_approx/3(FittingParameters), Lqq_approx1/3(FittingParameters)

== system uz_pmsm_model_old_commit/Current_Controller1/Reglernachführung ==
  Flag : Inport
  Ldd : Inport  Port=2
  Lqq : Inport  Port=3
  Constant : Constant  Value=1/(2*tau_sum)
  Constant1 : Constant  Value=R_1
  Constant2 : Constant  Value=L_d
  Constant3 : Constant  Value=L_q
  Product : Product
  Product1 : Product
  Product2 : Product
  Rate Transition1 : RateTransition  OutPortSampleTime=ts_regler
  Rate Transition12 : RateTransition  OutPortSampleTime=ts_regler
  Switch : Switch  Criteria=u2 > Threshold  SaturateOnIntegerOverflow=off  InputSameDT=off  OutDataTypeStr=Inherit: Same as first input
  Switch1 : Switch  Criteria=u2 > Threshold  SaturateOnIntegerOverflow=off  InputSameDT=off  OutDataTypeStr=Inherit: Same as first input
  K_p_d : Outport
  K_p_q : Outport  Port=2
  K_I : Outport  Port=3
  wires:
  Constant/1 -> Rate Transition12/1
  Product/1 -> K_p_d/1
  Product1/1 -> K_p_q/1
  Product2/1 -> K_I/1
  Rate Transition12/1 -> Product2/1, Product1/1, Product/2  "id_regler"
  Rate Transition1/1 -> Product2/2  "id_regler"
  Flag/1 -> Switch/2, Switch1/2
  Constant2/1 -> Switch/3
  Switch/1 -> Product/1
  Constant3/1 -> Switch1/3
  Switch1/1 -> Product1/2
  Ldd/1 -> Switch/1  "Ldd"
  Lqq/1 -> Switch1/1  "Lqq"
  Constant1/1 -> Rate Transition1/1  "u_q"

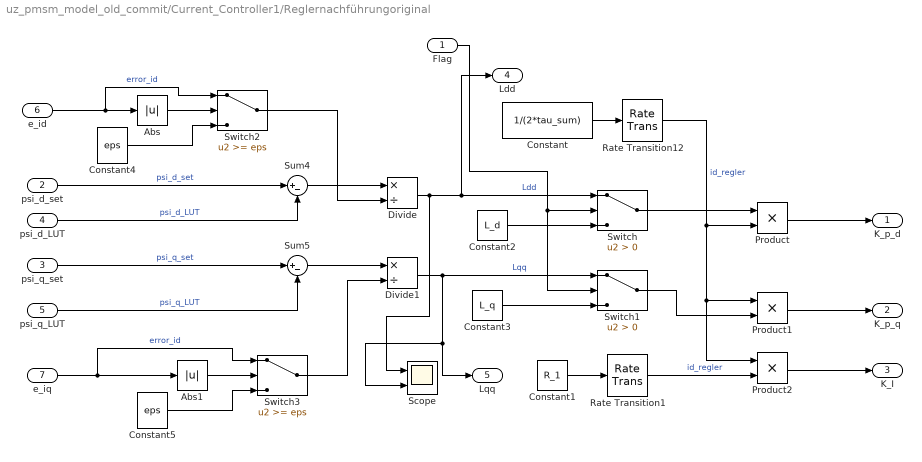
== system uz_pmsm_model_old_commit/Current_Controller1/Reglernachführungoriginal ==
  Flag : Inport
  psi_d_set : Inport  Port=2
  psi_q_set : Inport  Port=3
  psi_d_LUT : Inport  Port=4
  psi_q_LUT : Inport  Port=5
  e_id : Inport  Port=6
  e_iq : Inport  Port=7
  Abs : Abs  SaturateOnIntegerOverflow=off
  Abs1 : Abs  SaturateOnIntegerOverflow=off
  Constant : Constant  Value=1/(2*tau_sum)
  Constant1 : Constant  Value=R_1
  Constant2 : Constant  Value=L_d
  Constant3 : Constant  Value=L_q
  Constant4 : Constant  Value=eps  SampleTime=ts_regler
  Constant5 : Constant  Value=eps  SampleTime=ts_regler
  Divide : Product  Inputs=*/
  Divide1 : Product  Inputs=*/
  Product : Product
  Product1 : Product
  Product2 : Product
  Rate Transition1 : RateTransition  OutPortSampleTime=ts_regler
  Rate Transition12 : RateTransition  OutPortSampleTime=ts_regler
  Scope : Scope  NumInputPorts=2
  Sum4 : Sum  Inputs=|+-
  Sum5 : Sum  Inputs=|+-
  Switch : Switch  Criteria=u2 > Threshold  SaturateOnIntegerOverflow=off  InputSameDT=off
  Switch1 : Switch  Criteria=u2 > Threshold  SaturateOnIntegerOverflow=off  InputSameDT=off
  Switch2 : Switch  Threshold=eps  SaturateOnIntegerOverflow=off  InputSameDT=off
  Switch3 : Switch  Threshold=eps  SaturateOnIntegerOverflow=off  InputSameDT=off
  K_p_d : Outport
  K_p_q : Outport  Port=2
  K_I : Outport  Port=3
  Ldd : Outport  Port=4
  Lqq : Outport  Port=5
  wires:
  Constant/1 -> Rate Transition12/1
  Product/1 -> K_p_d/1
  Product1/1 -> K_p_q/1
  Product2/1 -> K_I/1
  Constant1/1 -> Rate Transition1/1
  Rate Transition12/1 -> Product2/1, Product1/1, Product/2  "id_regler"
  Rate Transition1/1 -> Product2/2  "id_regler"
  Flag/1 -> Switch/2, Switch1/2
  Constant2/1 -> Switch/3
  Switch/1 -> Product/1
  Constant3/1 -> Switch1/3
  Switch1/1 -> Product1/2
  Sum4/1 -> Divide/1
  psi_q_LUT/1 -> Sum5/2  "psi_q_LUT"
  Sum5/1 -> Divide1/1
  psi_d_LUT/1 -> Sum4/2  "psi_d_LUT"
  psi_d_set/1 -> Sum4/1  "psi_d_set"
  psi_q_set/1 -> Sum5/1  "psi_q_set"
  Divide/1 -> Scope/1, Ldd/1, Switch/1  "Ldd"
  Divide1/1 -> Scope/2, Lqq/1, Switch1/1  "Lqq"
  e_id/1 -> Switch2/1, Abs/1  "error_id"
  Constant4/1 -> Switch2/3
  Abs/1 -> Switch2/2
  Switch2/1 -> Divide/2
  e_iq/1 -> Switch3/1, Abs1/1  "error_id"
  Switch3/1 -> Divide1/2
  Abs1/1 -> Switch3/2
  Constant5/1 -> Switch3/3

== system uz_pmsm_model_old_commit/Current_Controller_With_FluxMaps_OLD1/Entkopplung_flags ==
  u_d_static : Inport
  u_q_static : Inport  Port=2
  u_d_praed : Inport  Port=3
  u_q_praed : Inport  Port=4
  u_d_lin : Inport  Port=5
  u_q_lin : Inport  Port=6
  u_d_dyn : Inport  Port=7
  u_q_dyn : Inport  Port=8
  0 : Constant  Value=0
  Switch{1..8} (8 alike) : Switch  Criteria=u2 > Threshold  SaturateOnIntegerOverflow=off  InputSameDT=off
  entkopplung_dynamic : Constant  Value=entkopplung_dynamic
  entkopplung_linear : Constant  Value=entkopplung_linear
  entkopplung_preadiktion : Constant  Value=praediktion_entkopplung_nonlinear
  entkopplung_static : Constant  Value=entkopplung_static
  u_d_entk : Outport
  u_q_entk : Outport  Port=2
  wires:
  Switch3/1 -> u_d_entk/1
  Switch4/1 -> Switch2/3
  entkopplung_preadiktion/1 -> Switch2/2, Switch3/2
  Switch1/1 -> Switch3/3
  u_d_praed/1 -> Switch3/1
  Switch2/1 -> u_q_entk/1
  u_q_praed/1 -> Switch2/1
  entkopplung_static/1 -> Switch4/2, Switch1/2
  u_d_static/1 -> Switch1/1
  u_d_lin/1 -> Switch5/1
  Switch5/1 -> Switch1/3
  entkopplung_linear/1 -> Switch6/2, Switch5/2
  entkopplung_dynamic/1 -> Switch8/2, Switch7/2
  0/1 -> Switch8/3, Switch7/3
  Switch6/1 -> Switch4/3
  u_q_static/1 -> Switch4/1
  u_q_lin/1 -> Switch6/1
  u_d_dyn/1 -> Switch7/1
  Switch8/1 -> Switch6/3
  u_q_dyn/1 -> Switch8/1
  Switch7/1 -> Switch5/3

== system uz_pmsm_model_old_commit/Current_Controller_With_FluxMaps_OLD1/Entkopplungen ==
  u_q : Inport
  u_d : Inport  Port=2
  uq : Inport  Port=3
  ud : Inport  Port=4
  i_d : Inport  Port=5
  psi_d_LUT : Inport  Port=6
  psi_q_LUT : Inport  Port=7
  Ldq_LUT : Inport  Port=8
  Lqd_LUT : Inport  Port=9
  i_q : Inport  Port=10
  omega_m : Inport  Port=11
  Lineare_Entkopplung : Subsystem
  decoupling_praediktion : Subsystem
  dynamic_nonlinear_entkopplung1 : Subsystem
  static_nonlinear_entkopplung : Subsystem
  u_d_static : Outport
  u_q_static : Outport  Port=2
  u_d_prae : Outport  Port=3
  u_q_prae : Outport  Port=4
  u_d_lin : Outport  Port=5
  u_q_lin : Outport  Port=6
  u_d_dyn : Outport  Port=7
  u_q_dyn1 : Outport  Port=8
  wires:
  psi_d_LUT/1 -> static_nonlinear_entkopplung/1(psi_d), dynamic_nonlinear_entkopplung1/3(psi_d), decoupling_praediktion/9(psi_d)
  omega_m/1 -> dynamic_nonlinear_entkopplung1/7(omega_m), Lineare_Entkopplung/3(omega_m), static_nonlinear_entkopplung/3(omega_m), decoupling_praediktion/5(omega_m)
  psi_q_LUT/1 -> dynamic_nonlinear_entkopplung1/4(psi_q), decoupling_praediktion/8(psi_q), static_nonlinear_entkopplung/2(psi_q)
  u_q/1 -> decoupling_praediktion/4(u_q_1)
  i_d/1 -> dynamic_nonlinear_entkopplung1/1(i_d), Lineare_Entkopplung/1(i_d), decoupling_praediktion/1(i_d)
  i_q/1 -> dynamic_nonlinear_entkopplung1/2(i_q), Lineare_Entkopplung/2(i_q), decoupling_praediktion/3(i_q)
  ud/1 -> decoupling_praediktion/6(u_d_k)
  uq/1 -> decoupling_praediktion/7(u_q_k)
  u_d/1 -> decoupling_praediktion/2(u_d_1)
  static_nonlinear_entkopplung/1(u_d) -> u_d_static/1
  Lineare_Entkopplung/1(u_d) -> u_d_lin/1
  static_nonlinear_entkopplung/2(u_q) -> u_q_static/1
  decoupling_praediktion/1(u_d_entk) -> u_d_prae/1
  Lineare_Entkopplung/2(u_q) -> u_q_lin/1
  decoupling_praediktion/2(u_q_entk) -> u_q_prae/1
  dynamic_nonlinear_entkopplung1/1(u_d) -> u_d_dyn/1
  dynamic_nonlinear_entkopplung1/2(u_q) -> u_q_dyn1/1
  Ldq_LUT/1 -> dynamic_nonlinear_entkopplung1/5(Ldq_LUT)
  Lqd_LUT/1 -> dynamic_nonlinear_entkopplung1/6(Lqd_LUT)

== system uz_pmsm_model_old_commit/Current_Controller_With_FluxMaps_OLD1/Psi_d_q ==
  I_d_set : Inport
  I_d : Inport  Port=2
  I_q_set : Inport  Port=3
  I_q : Inport  Port=4
  Flux_d Lookup Table : Lookup_n-D  BreakpointsForDimension1=d_current_d_Flux  BreakpointsForDimension2=q_current_d_Flux  BreakpointsForDimension3=[5, 7]  Table=Flux_d  InternalRulePriority=Speed  RndMeth=Simplest
      settings: InputPortMap=u0,u1
  Flux_d Lookup Table1 : Lookup_n-D  BreakpointsForDimension1=d_current_d_Flux  BreakpointsForDimension2=q_current_d_Flux  BreakpointsForDimension3=[5, 7]  Table=Flux_d  InternalRulePriority=Speed  RndMeth=Simplest
      settings: InputPortMap=u0,u1
  Flux_q Lookup Table1 : Lookup_n-D  BreakpointsForDimension1=d_current_q_Flux  BreakpointsForDimension2=q_current_q_Flux  BreakpointsForDimension3=[5, 7]  Table=Flux_q  InternalRulePriority=Speed  RndMeth=Simplest
      settings: InputPortMap=u0,u1
  Flux_q Lookup Table2 : Lookup_n-D  BreakpointsForDimension1=d_current_q_Flux  BreakpointsForDimension2=q_current_q_Flux  BreakpointsForDimension3=[5, 7]  Table=Flux_q  InternalRulePriority=Speed  RndMeth=Simplest
      settings: InputPortMap=u0,u1
  Ldq Lookup Table : Lookup_n-D  BreakpointsForDimension1=d_current_q_Flux  BreakpointsForDimension2=q_current_q_Flux  BreakpointsForDimension3=[5, 7]  Table=Ldq  ExtrapMethod=Clip  UseLastTableValue=on  InternalRulePriority=Speed  OutDataTypeStr=Inherit: Inherit from 'Table data'  RndMeth=Simplest
      settings: InputPortMap=u0,u1
  Lqd Lookup Table1 : Lookup_n-D  BreakpointsForDimension1=d_current_q_Flux  BreakpointsForDimension2=q_current_q_Flux  BreakpointsForDimension3=[5, 7]  Table=Ldq  ExtrapMethod=Clip  UseLastTableValue=on  InternalRulePriority=Speed  OutDataTypeStr=Inherit: Inherit from 'Table data'  RndMeth=Simplest
      settings: InputPortMap=u0,u1
  Scope : Scope  NumInputPorts=4
  psi_d_set : Outport
  psi_q_set : Outport  Port=2
  psi_d_LUT : Outport  Port=3
  psi_q_LUT : Outport  Port=4
  Ldq_LUT : Outport  Port=5
  Lqd_LUT : Outport  Port=6
  wires:
  I_d_set/1 -> Scope/1, Flux_d Lookup Table1/1
  I_q_set/1 -> Scope/2, Flux_q Lookup Table2/2
  Flux_d Lookup Table1/1 -> psi_d_set/1  "psi_d_set"
  Flux_q Lookup Table2/1 -> psi_q_set/1  "psi_q_set"
  Flux_d Lookup Table/1 -> psi_d_LUT/1  "psi_d_controller"
  Flux_q Lookup Table1/1 -> psi_q_LUT/1  "psi_q_controller"
  Ldq Lookup Table/1 -> Ldq_LUT/1  "Ldq_Karte"
  Lqd Lookup Table1/1 -> Lqd_LUT/1  "Ldq_Karte"
  I_d/1 -> Scope/3, Flux_q Lookup Table2/1, Lqd Lookup Table1/1, Ldq Lookup Table/1, Flux_q Lookup Table1/1, Flux_d Lookup Table/1
  I_q/1 -> Scope/4, Lqd Lookup Table1/2, Ldq Lookup Table/2, Flux_q Lookup Table1/2, Flux_d Lookup Table1/2, Flux_d Lookup Table/2

== system uz_pmsm_model_old_commit/Current_Controller_With_FluxMaps_OLD1/Psi_d_q1 ==
  I_d_set : Inport
  I_d : Inport  Port=2
  I_q_set : Inport  Port=3
  I_q : Inport  Port=4
  Flux_d Lookup Table : Lookup_n-D  BreakpointsForDimension1=d_current_d_Flux  BreakpointsForDimension2=q_current_d_Flux  BreakpointsForDimension3=[5, 7]  Table=Flux_d  InternalRulePriority=Speed  RndMeth=Simplest
      settings: InputPortMap=u0,u1
  Flux_d Lookup Table1 : Lookup_n-D  BreakpointsForDimension1=d_current_d_Flux  BreakpointsForDimension2=q_current_d_Flux  BreakpointsForDimension3=[5, 7]  Table=Flux_d  InternalRulePriority=Speed  RndMeth=Simplest
      settings: InputPortMap=u0,u1
  Flux_q Lookup Table1 : Lookup_n-D  BreakpointsForDimension1=d_current_q_Flux  BreakpointsForDimension2=q_current_q_Flux  BreakpointsForDimension3=[5, 7]  Table=Flux_q  InternalRulePriority=Speed  RndMeth=Simplest
      settings: InputPortMap=u0,u1
  Flux_q Lookup Table2 : Lookup_n-D  BreakpointsForDimension1=d_current_q_Flux  BreakpointsForDimension2=q_current_q_Flux  BreakpointsForDimension3=[5, 7]  Table=Flux_q  InternalRulePriority=Speed  RndMeth=Simplest
      settings: InputPortMap=u0,u1
  Ldq Lookup Table : Lookup_n-D  BreakpointsForDimension1=d_current_q_Flux  BreakpointsForDimension2=q_current_q_Flux  BreakpointsForDimension3=[5, 7]  Table=Ldq  ExtrapMethod=Clip  UseLastTableValue=on  InternalRulePriority=Speed  OutDataTypeStr=Inherit: Inherit from 'Table data'  RndMeth=Simplest
      settings: InputPortMap=u0,u1
  Lqd Lookup Table1 : Lookup_n-D  BreakpointsForDimension1=d_current_q_Flux  BreakpointsForDimension2=q_current_q_Flux  BreakpointsForDimension3=[5, 7]  Table=Ldq  ExtrapMethod=Clip  UseLastTableValue=on  InternalRulePriority=Speed  OutDataTypeStr=Inherit: Inherit from 'Table data'  RndMeth=Simplest
      settings: InputPortMap=u0,u1
  psi_d_set : Outport
  psi_q_set : Outport  Port=2
  psi_d_LUT : Outport  Port=3
  psi_q_LUT : Outport  Port=4
  Ldq_LUT : Outport  Port=5
  Lqd_LUT : Outport  Port=6
  wires:
  I_d_set/1 -> Flux_d Lookup Table1/1
  I_q_set/1 -> Flux_q Lookup Table2/2
  Flux_d Lookup Table1/1 -> psi_d_set/1  "psi_d_set"
  Flux_q Lookup Table2/1 -> psi_q_set/1  "psi_q_set"
  Flux_d Lookup Table/1 -> psi_d_LUT/1  "psi_d_controller"
  Flux_q Lookup Table1/1 -> psi_q_LUT/1  "psi_q_controller"
  Ldq Lookup Table/1 -> Ldq_LUT/1  "Ldq_Karte"
  Lqd Lookup Table1/1 -> Lqd_LUT/1  "Ldq_Karte"
  I_d/1 -> Flux_q Lookup Table2/1, Lqd Lookup Table1/1, Ldq Lookup Table/1, Flux_q Lookup Table1/1, Flux_d Lookup Table/1
  I_q/1 -> Lqd Lookup Table1/2, Ldq Lookup Table/2, Flux_q Lookup Table1/2, Flux_d Lookup Table1/2, Flux_d Lookup Table/2
